simulink model "MTDC_MODEL"  (R2021a)
settings: Solver=ode1  StartTime=0.0  StopTime=3  FixedStep=2e-5  MaxStep=1e-5  RelTol=1e-5  EnableMultiTasking=on
InitFcn:
  | tau_iac=ts_G_iac/4;                                         %Current loop speed
  | wAC=1/tau_iac;                                              %Frequency
  | L1AC=wAC/s;                                                 %Open loop IMC (L) transfer function to obtain a first order after closing the loop
  | Kp_AC=wAC*(Lg_1+La_1/2);                                    %Proportional constant of the controller
  | Ki_AC=wAC*(Rg_1+Ra_1/2);                                    %Integral constant of the controller
  | C_IMC_AC=(Kp_AC*s+Ki_AC)/s;                                 %IMC designed PI controller transfer function
  | TAC=minreal((C_IMC_AC)*G_iac/(1+(C_IMC_AC)*G_iac));         %Closed loop transfer function
  | 
  | tau_Pac=ts_G_P/4;
  | D = TAC*U_ll1;
  | [C_pi,info] = pidtune(D,'PI',1/tau_Pac);
  | Ki_P = C_pi.Ki;
  | 
  | tau_Qac=ts_G_Q/4;
  | [C_piq,info] = pidtune(D,'PI',1/tau_Qac);
  | Ki_Q = C_piq.Ki;
  | 
  | 
  | tau_isum=ts_G_isum/4;                                        %Current loop speed
  | wsum=1/tau_isum;                                             %Frequency
  | L1AC=wsum/s;                                                 %Open loop IMC (L) transfer function to obtain a first order after closing the loop
  | Kp_sum=wsum*(2*La_1);                                        %Proportional constant of the controller
  | Ki_sum=wsum*(2*Ra_1);                                        %Integral constant of the controller
  | C_IMC_sum=(Kp_sum*s+Ki_sum)/s;                               %IMC designed PI controller transfer function
  | 
  | Kp_sum_PR = wc*(2*La_1);
  | Ki_sum_PR = wc*(2*Ra_1);
  | PR = (Kp_sum_PR*s^2 + 2*wc*(Kp_sum_PR+Ki_sum_PR)*s +Kp_sum_PR*w0^2)/(s^2+2*wc*s+w0^2);
  | 
  | 
  | %Energy reference for a converter arm (sum of all the submodule energies)
  | ArmEnergyRef=1/2*Carm*ArmVoltageRef^2;                      %Energy reference for a converter leg
  | LegEnergy=ArmEnergyRef*2;                                   %References for the controllers (DC side)
  | TotalEnergyRef=ArmEnergyRef*6;                              %Reference of the total energy of the converter
  | EnergyDiffabRef=0;                                          %Reference for the energy difference between legs a and b
  | EnergyDiffacRef=0;                                          %Reference for the energy difference between legs b and c
  | 
  | %References for the controllers (AC side)
  | EnergyDiffUpLowRefa=0;                                      %Reference for the energy difference upper and lower arms of phase a
  | EnergyDiffUpLowRefb=0;                                      %Reference for the energy difference upper and lower arms of phase b
  | EnergyDiffUpLowRefc=0;                                      %Reference for the energy difference upper and lower arms of phase c
  |                                                             %Controller design
  | Kpenergy=50;                                                %Proportional gain
  | Kienergy=20;                                                %Integral gain
  | 
  | Kpenergyt=50;                                               %Proportional gain
  | Kienergyt=20;                                               %Integral gain
  | 
  | Q=3;
  | wn=50*2*pi;                                                 %Frequency to eliminate 50 Hz
  | N_50 = tf([1 0 wn^2],[1 2*wn/Q wn^2]);                       %Notch filter 1 design
  | wn=100*2*pi;                                                %Frequency to eliminate 100 Hz
  | N_100 = tf([1 0 wn^2],[1 2*wn/Q wn^2]);                      %Notch filter 2 design
  | Notch=N_50*N_100;                                            %Combination of both notch filters
  | 
  | Ibasedc1= 1000e6/640e3;                 %Nominal current peak DC
  | IsaturationinnerDC1=1.1*Ibasedc1/3;  %Saturation of the DC inner current
  | IsaturationinnerAC1=0.45*Ibasedc1/3; %0.45  %Saturation of the inner current (why edu used 10% - FYI I changed it to 45%)
  | 
  | 
  | ... (+30 lines)
values from neighbouring files (symbols this model uses):
  ArmVoltageRef = 640e3    (= 640000)    [MMC_PARAMETERS.m]
  Cap = 9.5e-3    (= 0.0095)    [MMC_PARAMETERS.m]
  Carm = Cap/N    (= 2.375e-05)    [MMC_PARAMETERS.m]
  f_grid = 50    [MMC_PARAMETERS.m]
  La_1 = 0.15*Zbase_1/2/pi/50    (= 0.0488923985178)    [MMC_PARAMETERS.m]
  Lg_1 = 0.18*Zbase_1/2/pi/50    (= 0.0586708782214)    [MMC_PARAMETERS.m]
  N = 400    [MMC_PARAMETERS.m]
  Ra_1 = 0.01*Zbase_1    (= 1.024)    [MMC_PARAMETERS.m]
  Rg_1 = 0.005*Zbase_1    (= 0.512)    [MMC_PARAMETERS.m]
  S_1 = 1000e6    (= 1000000000)    [MMC_PARAMETERS.m]
  U_ll1 = 320e3    (= 320000)    [MMC_PARAMETERS.m]
  Vdc = 640e3    (= 640000)    [MMC_PARAMETERS.m]
  Vpeak_d1 = U_pnpeak1    [MMC_PARAMETERS.m]
  w0 = 2*pi*50    (= 314.159265359)    [MMC_PARAMETERS.m]
undefined symbols (not defined in the file or in its folder): Kp_Pac, lenght
libraries: spsSeriesRLCBranchLib x80, spsCurrentMeasurementLib x64, spsControlledVoltageSourceLib x36, pid_lib x32, spsVoltageMeasurementLib x32, spsControlledCurrentSourceLib x24, spsParallelRLCBranchLib x20, spsGroundLib x10, powerlib_extras x4, spsDCVoltageSourceLib x4, spspowerguiLib x1
(part 2 of 9)

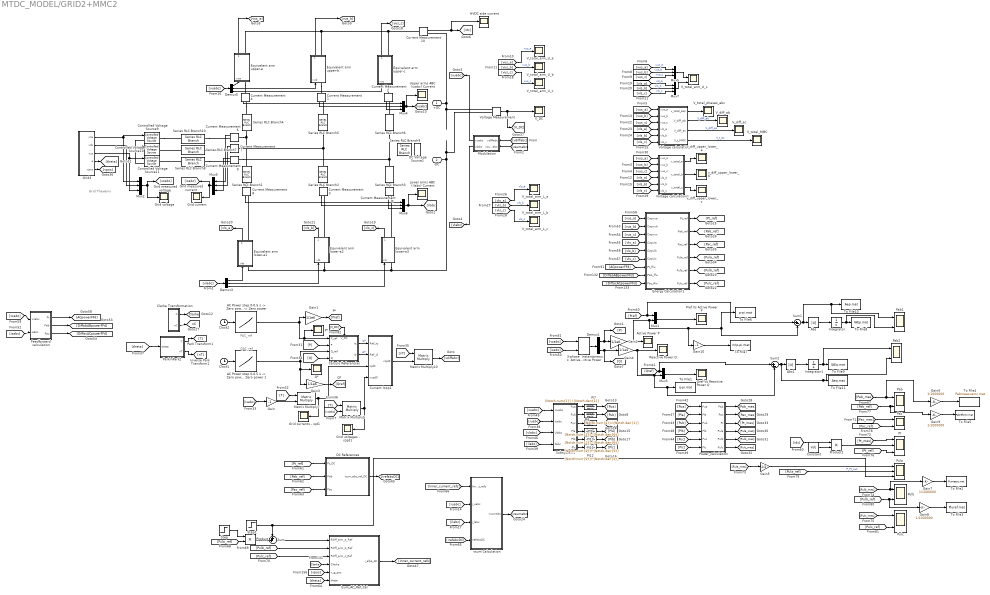
== system MTDC_MODEL/GRID2+MMC2 ==
  note: QAC_ref
  note: Grid Thevenin
  note: PAC_ref
  3-phase  Instantaneous  Active & Reactive Power : powerlib_extras/Measurements/3-phase  Instantaneous  Active & Reactive Power
      settings: SourceProductBaseCode=PS
  "AC Power step 0-0.5 s -> Zero power 0.5-2 s -> Active power injection 2 - 3 s -> Zero power " : Lookup_n-D  NumberOfTableDimensions=1  BreakpointsForDimension1=[0,0.5,2]  Table=[0,100e6,0]  InterpMethod=Flat  RndMeth=Simplest  InputSameDT=on
  "AC Power step 0-0.5 s -> Zero power 0.5-2 s -> Reactive power injection 2 - 3 s -> Zero power 1" : Lookup_n-D  NumberOfTableDimensions=1  BreakpointsForDimension1=[0,1,2]  Table=[0,5e6,0]  InterpMethod=Flat  RndMeth=Simplest  InputSameDT=on
  Abs : Abs
  Abs1 : Abs
  Active Power P : Scope
  Calculo Referencias : Subsystem
      settings: PortSchema="{\"entries\":[{\"content\":{\"sides\":[{\"content\":{\"connectorIds\":[\"In1\",\"In2\",\"In3\",\"In4\"]},\"type\":\"ConnectorPlacement.EquallySpacedRectSide\",\"uuid\":\"f5831c6a-58f5-4c55-8e24-523faf20dc0e\"},{\"content\":{\"connectorIds\":[\"Out1\",\"Out2\"],\"side\":\"RIGHT\"},\"type\":\"ConnectorPlacement.EquallySpacedRectSide\",\"uuid\":\"8e89a825-42f3-407f-8ce2-a529bb4d6e75\"},{\"content\":{\"connectorIds\":[\"In5\"],\"side\":\"TOP\"},\"type\":\"ConnectorPlacement.EquallySpacedRectSide\",\"uuid\":\"db0af466-562a-4a22-9801-d0efcc420c94\"},{\"content\":{\"connectorIds\":[],\"side\":\"BOTTOM\"},\"type\":\"ConnectorPlacement.EquallySpacedRectSide\",\"uuid\":\"e71aeab6-b02a-4177-93b6-e0e9fbfda2d5\"}]},\"type\":\"ConnectorPlacement.EquallySpacedConnector\",\"uuid\":\"54c33138-0c8b-4291-a3b0-05da54bcdffb\"}],\"packageUris\":[\"http://schema.mathworks.com/mf0/Connector/R2020b\"],\"version\":\"1.0\"}"
  "Clarke Transformation " : Subsystem
  Clock1 : Clock
  Clock2 : Clock
  Constant : Constant  Value=Vdc
  Controlled Voltage Source10 : spsControlledVoltageSourceLib/Controlled Voltage Source  Initialize=off  Source_Type=AC  Amplitude=0  Phase=0  Frequency=0  Measurements=None
  Controlled Voltage Source11 : spsControlledVoltageSourceLib/Controlled Voltage Source  Initialize=off  Source_Type=AC  Amplitude=0  Phase=0  Frequency=0  Measurements=None
  Controlled Voltage Source9 : spsControlledVoltageSourceLib/Controlled Voltage Source  Initialize=off  Source_Type=AC  Amplitude=0  Phase=0  Frequency=0  Measurements=None
  Current Measurement{1..10} (10 alike) : spsCurrentMeasurementLib/Current Measurement  PhasorSimulation=off  OutputType=Complex  PSBequivalent=0
  Current loop1 : Subsystem
  DC References : Subsystem
  DC Voltage Source1 : spsDCVoltageSourceLib/DC Voltage Source  Amplitude=Vdc  Measurements=None
  Demux1 : Demux  Outputs=2
  Demux3 : Demux  Outputs=3
  Demux5 : Demux  Outputs=3
  Energy Calculation1 : Subsystem
  Equivalent arm lower-a1 : Subsystem
  Equivalent arm lower-a2 : Subsystem
  Equivalent arm lower-a3 : Subsystem
  Equivalent arm upper-a : Subsystem
  Equivalent arm upper-b : Subsystem
  Equivalent arm upper-c : Subsystem
  Feedforward calculation : Subsystem
  Gain : Gain  Gain=-1
  Gain{1..4} (4 alike) : Gain  Gain=1/1e6
  Gain10 : Gain  Gain=-1
  Gain5 : Gain  Gain=-1/2
  Gain{6..9} (4 alike) : Gain  Gain=1/1000000
  Grid current : Scope
  Grid currents - iqd1 : Scope
  Grid voltage : Scope
  Grid voltages - vzqd1 : Scope
  Grid3 : Subsystem
  HVDC side current : Scope
  Integrator : Integrator
  Integrator1 : Integrator
  Isum_AC_Ref_Cal : Subsystem
  Lower arms ABC (ilabc) Current : Scope
  Matrix Multiply10 : Product  Multiplication=Matrix(*)
  Matrix Multiply5 : Product  Multiplication=Matrix(*)
  Matrix Multiply7 : Product  Multiplication=Matrix(*)
  Modulation : Subsystem
  Mux1 : Mux  Inputs=2
  Mux{2,4..7,9} (6 alike) : Mux  Inputs=3
  Mux3 : Mux  Inputs=2
  P* : Scope
  PI{7..12} (6 alike) : TransferFcn  Numerator=[Notch.num{1}]  Denominator=[Notch.den{1}]
  Pab : Scope  NumInputPorts=2
  Pab1 : Scope  NumInputPorts=2
  Pab2 : Scope  NumInputPorts=2
  Pac : Scope  NumInputPorts=2
  Park/nPark2 : Subsystem
  Power_calculation : Subsystem
  Pref Vs Active Power P : Scope
  Product : Product
  Product1 : Product
  Pt : Scope  NumInputPorts=3
  Pula : Scope  NumInputPorts=3
  Pulb : Scope  NumInputPorts=2
  Pulc : Scope  NumInputPorts=2
  Q* : Scope
  Qref Vs Reactive Power Q : Scope
  Reactive Power Q : Scope
  Series RLC Branch{1..6} (6 alike) : spsSeriesRLCBranchLib/Series RLC Branch  LConnTagsString=__new0  RConnTagsString=__new0  BranchType=RL  Resistance=Ra_1  Inductance=La_1  SetiL0=off  InitialCurrent=0  Capacitance=0  Setx0=off  InitialVoltage=0  Measurements=None
  Series RLC Branch10 : spsSeriesRLCBranchLib/Series RLC Branch  LConnTagsString=__new0  RConnTagsString=__new0  BranchType=RL  Resistance=Rg_1  Inductance=Lg_1  SetiL0=off  InitialCurrent=0  Capacitance=0  Setx0=off  InitialVoltage=0  Measurements=None
  Series RLC Branch7 : spsSeriesRLCBranchLib/Series RLC Branch  LConnTagsString=__new0  RConnTagsString=__new0  BranchType=RL  Resistance=Rg_1  Inductance=Lg_1  SetiL0=off  InitialCurrent=0  Capacitance=0  Setx0=off  InitialVoltage=0  Measurements=None
  Series RLC Branch8 : spsSeriesRLCBranchLib/Series RLC Branch  LConnTagsString=__new0  RConnTagsString=__new0  BranchType=RL  Resistance=Rg_1  Inductance=Lg_1  SetiL0=off  InitialCurrent=0  Capacitance=0  Setx0=off  InitialVoltage=0  Measurements=None
  Series RLC Branch9 : spsSeriesRLCBranchLib/Series RLC Branch  LConnTagsString=__new0  RConnTagsString=__new0  BranchType=C  Resistance=1  Inductance=1e-3  SetiL0=off  InitialCurrent=0  Capacitance=6*Carm  Setx0=off  InitialVoltage=0  Measurements=None
  Step : Step  Time=2.1  Before=1  After=0  SampleTime=0
  Step1 : Step  Time=2.1  After=-1e6  SampleTime=0
  Subsystem1 : Subsystem
  Sum : Sum  Inputs=++|
  Sum1 : Sum  Inputs=|+-
  Sum2 : Sum  Inputs=|+-
  To File1 : ToFile  Filename=q-pi.mat  MatrixName=qsmc  SaveFormat=Timeseries
  To File10 : ToFile  Filename=Aep.mat  MatrixName=Aep  SaveFormat=Timeseries
  To File11 : ToFile  Filename=Aeq.mat  MatrixName=Aeq  SaveFormat=Timeseries
  To File2 : ToFile  Filename=Plumeasu.mat  MatrixName=ans7  SaveFormat=Timeseries
  To File3 : ToFile  Filename=Pluref.mat  MatrixName=ans8  SaveFormat=Timeseries
  To File4 : ToFile  Filename=Pabmeasusmc.mat  MatrixName=ans0002  SaveFormat=Timeseries
  To File5 : ToFile  Filename=Pabrefsmc.mat  MatrixName=ans0001  SaveFormat=Timeseries
  To File6 : ToFile  Filename=p-pi.mat  MatrixName=psmc  SaveFormat=Timeseries
  To File7 : ToFile  Filename=nnp-pi.mat  MatrixName=ans00007  SaveFormat=Timeseries
  To File8 : ToFile  Filename=IAEp.mat  MatrixName=IAEp  SaveFormat=Timeseries
  To File9 : ToFile  Filename=IAEq.mat  MatrixName=IAEq  SaveFormat=Timeseries
  Upper arms ABC (iuabc) Current : Scope
  V_DC : Scope
  V_diff_ab : Scope
  V_diff_ac : Scope
  V_total_MMC : Scope
  V_total_arm_L_a : Scope
  V_total_arm_L_b : Scope
  V_total_arm_L_c : Scope
  V_total_arm_U_L : Scope  NumInputPorts=2
  V_total_arm_U_a : Scope
  V_total_arm_U_b : Scope
  V_total_arm_U_c : Scope
  V_total_phases_abc : Scope
  Voltage Measurement : spsVoltageMeasurementLib/Voltage Measurement  PhasorSimulation=off  OutputType=Complex  PSBequivalent=0
  Voltage calculation : Subsystem
  Voltage calculation1 : Subsystem
  v_diff_upper_lower_a : Scope
  v_diff_upper_lower_b : Scope
  v_diff_upper_lower_c : Scope
  vsum Calculation : Subsystem
  +DC : PMIOPort  Side=Left
  -DC : PMIOPort  Port=2  Side=Left
  tag scope: Clarke=global, nC=global
  wires:
  [V_DC] -> Calculo Referencias/5(V_DC)
  Current Measurement3/1 -> Mux6/2
  [vus_b] -> Energy Calculation1/2(Capvub)
  Energy Calculation1/2(Pab_ref) -> [Pab_ref]
  Voltage calculation1/2(v_total_b) -> v_diff_upper_lower_b/1
  [vus_a] -> Energy Calculation1/1(Capvua)
  Subsystem1/2(Pub) -> PI8/1
  [vls_b] -> Energy Calculation1/5(Capvlb)
  Gain1/1 -> [Pref]
  Current Measurement9/1 -> Mux9/3
  [vls_c] -> V_total_arm_L_c/1  "vls_c"
  Subsystem1/3(Puc) -> PI9/1
  [Pua] -> Power_calculation/1(Pua)
  [vdiffabc] -> Modulation/1(vdiffabc)
  [vzabc] -> 3-phase  Instantaneous  Active & Reactive Power/1
  Current Measurement2/1 -> Mux4/3
  Equivalent arm upper-a/1(v_sum_ua) -> [vus_a]
  [Plc] -> Power_calculation/6(Plc)
  [isabc] -> 3-phase  Instantaneous  Active & Reactive Power/2
  Matrix Multiply10/1 -> [vdiffabc]
  Mux6/1 -> Lower arms ABC (ilabc) Current/1, [ilabc]
  [theta] -> Park/nPark2/1(theta)
  [vls_a] -> Voltage calculation/4(vls_a)
  [P] -> Calculo Referencias/2(P)
  Park/nPark2/2("nT ") -> [nT]
  [nT] -> Matrix Multiply10/1
  Equivalent arm upper-c/1(v_sum_uc) -> [vus_c]
  Gain3/1 -> [Qref]
  Modulation/2(vlabc) -> [vlabc]
  [T] -> Matrix Multiply5/1
  Calculo Referencias/2(id) -> Current loop1/2(Ref_id)  "id*"
  Park/nPark2/1(T) -> [T]
  Voltage calculation/4(V_t_MMC) -> V_total_MMC/1  "V_t_ac"
  [Qref] -> Sum2/1, Mux3/1
  Gain2/1 -> Gain10/1, To File6/1, Sum1/2, Mux1/2, Active Power P/1
  Grid3/1(vza) -> Controlled Voltage Source9/1, Mux2/1
  Current loop1/1(vlqd0) -> Matrix Multiply10/2
  Mux2/1 -> [vzabc], Grid voltage/1
  Equivalent arm lower-a2/1(v_sum_lb) -> [vls_b]
  "AC Power step 0-0.5 s -> Zero power 0.5-2 s -> Reactive power injection 2 - 3 s -> Zero power 1"/1 -> Calculo Referencias/3(Q_ref), Gain3/1, Q*/1
  Equivalent arm lower-a1/1(v_sum_la) -> [vls_a]
  [vus_c] -> V_total_arm_U_c/1  "vus_c"
  [vus_c] -> Mux5/3  "vus_c"
  Voltage calculation/3(V_diff_ac) -> V_diff_ac/1  "V_diff_ac"
  [vus_b] -> V_total_arm_U_b/1  "vus_b"
  Mux3/1 -> Qref Vs Reactive Power Q/1
  [vus_b] -> Mux5/2  "vus_b"
  [vus_c] -> Voltage calculation/3(vus_c)
  [isabc] -> Gain/1
  [vls_b] -> V_total_arm_L_b/1  "vls_b"
  Equivalent arm upper-b/1(v_sum_ub) -> [vus_b]
  [vls_b] -> Mux7/2  "vls_b"
  [vls_a] -> Mux7/1  "vls_a"
  Voltage calculation1/1(v_total_a) -> v_diff_upper_lower_a/1
  [vls_c] -> Voltage calculation/6(vls_c)
  [vus_b] -> Voltage calculation1/2(vus_b)
  [vls_b] -> Voltage calculation1/5(vls_b)
  Constant/1 -> Product1/2
  Demux3/2 -> Equivalent arm lower-a2/1(vlb)
  Clock2/1 -> "AC Power step 0-0.5 s -> Zero power 0.5-2 s -> Active power injection 2 - 3 s -> Zero power "/1
  Matrix Multiply7/1 -> Current loop1/3(iqd0), Grid currents - iqd1/1
  Clock1/1 -> "AC Power step 0-0.5 s -> Zero power 0.5-2 s -> Reactive power injection 2 - 3 s -> Zero power 1"/1
  [vlabc] -> Subsystem1/3(Ulabc)
  [vus_a] -> Mux5/1  "vus_a"
  Gain/1 -> Matrix Multiply7/2
  [vpos] -> Isum_AC_Ref_Cal/5(v_g_pos)
  [Pula_ref] -> Product/2
  Step1/1 -> Pula/3, Sum/1
  Product1/1 -> Pt/2
  [ACpowerFFd] -> Energy Calculation1/7(Pt_ffw)
  [idc] -> Product1/1
  Power_calculation/3(Pt) -> [Pt_mes]
  [DiffabABpowerFFd] -> Energy Calculation1/8(Pab_ffw)
  [vls_a] -> Voltage calculation1/4(vls_a)
  [vus_c] -> Energy Calculation1/3(Capvuc)
  Subsystem1/1(Pua) -> PI7/1
  [Pula_ref] -> Pula/2  "P_PI_out"
  [vls_c] -> Energy Calculation1/6(Capvlc)
  [irefabcDC] -> vsum Calculation/4(irefabcDC)
  [vus_a] -> Voltage calculation1/1(vus_a)
  [Pula_mes] -> Gain5/1
  Mux1/1 -> Pref Vs Active Power P/1
  PI11/1 -> [Plb]
  DC References/1(isum_abc_ref_DC) -> [irefabcDC]
  [Pac_ref] -> DC References/3(Pac)
  Demux1/1 -> [P], Gain2/1
  Step/1 -> Product/1
  [Pub] -> Power_calculation/3(Pub)
  [Pac_mes] -> Pac/1
  [T] -> Matrix Multiply7/1
  Feedforward calculation/2(Pab) -> [DiffabABpowerFFd]
  Voltage Measurement/1 -> [V_DC], V_DC/1
  [vsumabc] -> Modulation/2(vsumabc)
  vsum Calculation/1(vsumabc) -> [vsumabc]
  Power_calculation/2(Pac) -> [Pac_mes]
  PI12/1 -> [Plc]
  [Puc] -> Power_calculation/5(Puc)
  Calculo Referencias/1(iq) -> Current loop1/1(Ref_iq)  "iq*"
  Mux7/1 -> V_total_arm_U_L/2
  Product/1 -> Sum/2
  Modulation/1(vuabc) -> [vuabc]
  Voltage calculation/1(v_total_abc) -> V_total_phases_abc/1
  [vus_a] -> V_total_arm_U_a/1  "vus_a"
  Sum/1 -> Isum_AC_Ref_Cal/1(Pdiff_arm_a_Ref)
  [Pab_ref] -> DC References/2(Pab)
  Power_calculation/5(Pulb) -> [Pulb_mes]
  [Pt_ref] -> Pt/3
  [vus_c] -> Voltage calculation1/3(vus_c)
  [Pref] -> Sum1/1, Mux1/1
  [Pulb_mes] -> Gain7/1, Pulb/1
  PI9/1 -> [Puc]
  Gain4/1 -> Sum2/2, To File1/1, Mux3/2, Reactive Power Q/1
  [vzabc] -> Matrix Multiply5/2
  Energy Calculation1/4(Pula_ref) -> [Pula_ref]
  PI10/1 -> [Pla]
  Power_calculation/6(Pulc) -> [Pulc_mes]
  Gain5/1 -> Pula/1
  Mux5/1 -> V_total_arm_U_L/1
  [Pulc_ref] -> Pulc/2
  [Plb] -> Power_calculation/4(Plb)
  Current Measurement7/1 -> Mux9/2
  PI8/1 -> [Pub]
  "AC Power step 0-0.5 s -> Zero power 0.5-2 s -> Active power injection 2 - 3 s -> Zero power "/1 -> P*/1, Calculo Referencias/1(P_ref), Gain1/1
  [Pulc_mes] -> Pulc/1
  Power_calculation/1(Pab) -> [Pab_mes]
  "Clarke Transformation "/2("nC ") -> [nC]
  Demux5/3 -> Equivalent arm upper-c/1(vuc)
  Energy Calculation1/3(Pac_ref) -> [Pac_ref]
  Mux4/1 -> Upper arms ABC (iuabc) Current/1, [iuabc]
  [Pac_ref] -> Pac/2
  [vls_c] -> Mux7/3  "vls_c"
  Subsystem1/5(Plb) -> PI11/1
  Matrix Multiply5/1 -> Grid voltages - vzqd1/1, Current loop1/4(vzqd0)
  [Pab_ref] -> Gain9/1, Pab/2
  Demux5/1 -> Equivalent arm upper-a/1(vua)
  Grid3/5(vpos) -> [vpos]
  Subsystem1/6(Plc) -> PI12/1
  [Pab_mes] -> Gain6/1, Pab/1
  Grid3/3(vzc) -> Controlled Voltage Source11/1, Mux2/3
  "Clarke Transformation "/1(C) -> [Clarke]
  Subsystem1/4(Pla) -> PI10/1
  [ilabc] -> vsum Calculation/3(i_labc)
  [iuabc] -> vsum Calculation/2(i_uabc)
  [DiffacACpowerFFd] -> Energy Calculation1/9(Pac_ffw)
  [isabc] -> Feedforward calculation/2(isabc)
  [Pulc_ref] -> Isum_AC_Ref_Cal/3(Pdiff_arm_c_Ref)
  [vus_a] -> Voltage calculation/1(vus_a)
  [theta] -> Isum_AC_Ref_Cal/6(theta)
  [vls_b] -> Voltage calculation/5(vls_b)
  [vzabc] -> Feedforward calculation/1(vzabc)
  [Clarke] -> Isum_AC_Ref_Cal/4(Clarke)
  Feedforward calculation/1(Pt) -> [ACpowerFFd]
  Mux9/1 -> [isabc], Grid current/1
  Feedforward calculation/3(Pac) -> [DiffacACpowerFFd]
  Voltage calculation/2(V_diff_ab) -> V_diff_ab/1  "V_diff_ab"
  Demux1/2 -> [Q], Gain4/1
  Current Measurement6/1 -> Mux9/1
  [ilabc] -> Subsystem1/4(Ilabc)
  [Pt_mes] -> Pt/1
  [vus_b] -> Voltage calculation/2(vus_b)
  [Pulb_ref] -> Gain8/1, Pulb/2
  [vlabc] -> Demux3/1
  Energy Calculation1/1(Pt_ref) -> [Pt_ref]
  Voltage calculation1/3(v_total_c) -> v_diff_upper_lower_c/1
  [vls_a] -> V_total_arm_L_a/1  "vls_a"
  Current Measurement4/1 -> Mux4/1
  [vuabc] -> Demux5/1
  Current Measurement1/1 -> Mux4/2
  [iuabc] -> Subsystem1/2(Iuabc)
  [vuabc] -> Subsystem1/1(Uuabc)
  Power_calculation/4(Pula) -> [Pula_mes]
  Demux5/2 -> Equivalent arm upper-b/1(vub)
  PI7/1 -> [Pua]
  [Q] -> Calculo Referencias/4(Q)
  Equivalent arm lower-a3/1(v_sum_lc) -> [vls_c]
  [vls_c] -> Voltage calculation1/6(vls_c)
  Demux3/3 -> Equivalent arm lower-a3/1(vlc)
  3-phase  Instantaneous  Active & Reactive Power/1 -> Demux1/1
  [Pt_ref] -> DC References/1(Pt_DC)
  Isum_AC_Ref_Cal/1(i_albe_AC) -> [Inner_current_refs]
  Energy Calculation1/6(Pulc_ref) -> [Pulc_ref]
  Current Measurement8/1 -> Mux6/1
  Energy Calculation1/5(Pulb_ref) -> [Pulb_ref]
  Current Measurement5/1 -> Mux6/3
  Demux3/1 -> Equivalent arm lower-a1/1(vla)
  [vls_a] -> Energy Calculation1/4(Capvla)
  Grid3/2(vzb) -> Controlled Voltage Source10/1, Mux2/2
  [Pulb_ref] -> Isum_AC_Ref_Cal/2(Pdiff_arm_b_Ref)
  Grid3/4(thetareal) -> [theta]
  [Pla] -> Power_calculation/2(Pla)
  Current Measurement10/1 -> HVDC side current/1, [idc]
  [Inner_current_refs] -> vsum Calculation/1(Inner_current_refs)
  Gain7/1 -> To File2/1
  Gain8/1 -> To File3/1
  Gain6/1 -> To File4/1
  Gain9/1 -> To File5/1
  Gain10/1 -> To File7/1
  Sum1/1 -> Pab1/1, To File10/1, Abs/1
  Abs/1 -> Integrator/1
  Integrator/1 -> Pab1/2, To File8/1
  Integrator1/1 -> Pab2/1, To File9/1
  Abs1/1 -> Integrator1/1
  Sum2/1 -> Pab2/2, To File11/1, Abs1/1
  connections:
  Equivalent arm lower-a1/LConn1 -- Equivalent arm lower-a2/LConn1 -- Voltage Measurement/LConn2 -- -DC/RConn1 -- Equivalent arm lower-a3/LConn1
  Current Measurement6/LConn1 -- Series RLC Branch4/RConn1 -- Series RLC Branch1/LConn1
  Voltage Measurement/LConn1 -- Current Measurement10/RConn1 -- +DC/RConn1
  Controlled Voltage Source10/LConn1 -- Controlled Voltage Source9/LConn1 -- Controlled Voltage Source11/LConn1
  Equivalent arm upper-a/RConn1 -- Current Measurement10/LConn1 -- Equivalent arm upper-c/RConn1 -- Equivalent arm upper-b/RConn1
  Current Measurement7/LConn1 -- Series RLC Branch5/RConn1 -- Series RLC Branch2/LConn1
  Current Measurement9/LConn1 -- Series RLC Branch6/RConn1 -- Series RLC Branch3/LConn1
  Series RLC Branch8/RConn1 -- Current Measurement9/RConn1
  Current Measurement4/RConn1 -- Series RLC Branch4/LConn1
  Series RLC Branch10/RConn1 -- Current Measurement6/RConn1
  Series RLC Branch7/LConn1 -- Controlled Voltage Source10/RConn1
  Equivalent arm lower-a1/RConn1 -- Current Measurement8/RConn1
  Equivalent arm lower-a3/RConn1 -- Current Measurement5/RConn1
  Series RLC Branch3/RConn1 -- Current Measurement5/LConn1
  Series RLC Branch8/LConn1 -- Controlled Voltage Source11/RConn1
  Series RLC Branch7/RConn1 -- Current Measurement7/RConn1
  Series RLC Branch1/RConn1 -- Current Measurement8/LConn1
  Series RLC Branch2/RConn1 -- Current Measurement3/LConn1
  Equivalent arm upper-c/LConn1 -- Current Measurement2/LConn1
  Series RLC Branch6/LConn1 -- Current Measurement2/RConn1
  Equivalent arm lower-a2/RConn1 -- Current Measurement3/RConn1
  Series RLC Branch5/LConn1 -- Current Measurement1/RConn1
  Controlled Voltage Source9/RConn1 -- Series RLC Branch10/LConn1
  Equivalent arm upper-a/LConn1 -- Current Measurement4/LConn1
  Equivalent arm upper-b/LConn1 -- Current Measurement1/LConn1

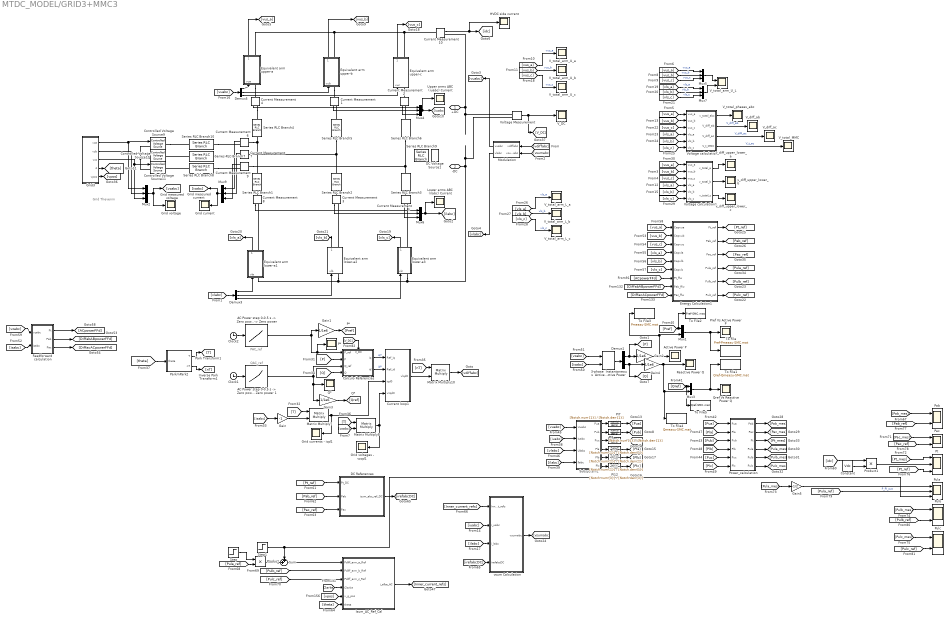
== system MTDC_MODEL/GRID3+MMC3 ==
  note: QAC_ref
  note: Grid Thevenin
  note: PAC_ref
  3-phase  Instantaneous  Active & Reactive Power : powerlib_extras/Measurements/3-phase  Instantaneous  Active & Reactive Power
      settings: SourceProductBaseCode=PS
  "AC Power step 0-0.5 s -> Zero power 0.5-2 s -> Active power injection 2 - 3 s -> Zero power " : Lookup_n-D  NumberOfTableDimensions=1  BreakpointsForDimension1=[0,0.5,2]  Table=[0,-100e6,0]  InterpMethod=Flat  RndMeth=Simplest  InputSameDT=on
  "AC Power step 0-0.5 s -> Zero power 0.5-2 s -> Reactive power injection 2 - 3 s -> Zero power 1" : Lookup_n-D  NumberOfTableDimensions=1  BreakpointsForDimension1=[0,1,2]  Table=[0,-5e6,0]  InterpMethod=Flat  RndMeth=Simplest  InputSameDT=on
  Active Power P : Scope
  Calculo Referencias : Subsystem
      settings: PortSchema="{\"entries\":[{\"content\":{\"sides\":[{\"content\":{\"connectorIds\":[\"In1\",\"In2\",\"In3\",\"In4\"]},\"type\":\"ConnectorPlacement.EquallySpacedRectSide\",\"uuid\":\"f5831c6a-58f5-4c55-8e24-523faf20dc0e\"},{\"content\":{\"connectorIds\":[\"Out1\",\"Out2\"],\"side\":\"RIGHT\"},\"type\":\"ConnectorPlacement.EquallySpacedRectSide\",\"uuid\":\"8e89a825-42f3-407f-8ce2-a529bb4d6e75\"},{\"content\":{\"connectorIds\":[\"In5\"],\"side\":\"TOP\"},\"type\":\"ConnectorPlacement.EquallySpacedRectSide\",\"uuid\":\"db0af466-562a-4a22-9801-d0efcc420c94\"},{\"content\":{\"connectorIds\":[],\"side\":\"BOTTOM\"},\"type\":\"ConnectorPlacement.EquallySpacedRectSide\",\"uuid\":\"e71aeab6-b02a-4177-93b6-e0e9fbfda2d5\"}]},\"type\":\"ConnectorPlacement.EquallySpacedConnector\",\"uuid\":\"54c33138-0c8b-4291-a3b0-05da54bcdffb\"}],\"packageUris\":[\"http://schema.mathworks.com/mf0/Connector/R2020b\"],\"version\":\"1.0\"}"
  Clock1 : Clock
  Clock2 : Clock
  Constant : Constant  Value=Vdc
  Controlled Voltage Source10 : spsControlledVoltageSourceLib/Controlled Voltage Source  Initialize=off  Source_Type=AC  Amplitude=0  Phase=0  Frequency=0  Measurements=None
  Controlled Voltage Source11 : spsControlledVoltageSourceLib/Controlled Voltage Source  Initialize=off  Source_Type=AC  Amplitude=0  Phase=0  Frequency=0  Measurements=None
  Controlled Voltage Source9 : spsControlledVoltageSourceLib/Controlled Voltage Source  Initialize=off  Source_Type=AC  Amplitude=0  Phase=0  Frequency=0  Measurements=None
  Current Measurement{1..10} (10 alike) : spsCurrentMeasurementLib/Current Measurement  PhasorSimulation=off  OutputType=Complex  PSBequivalent=0
  Current loop1 : Subsystem
  DC References : Subsystem
  DC Voltage Source1 : spsDCVoltageSourceLib/DC Voltage Source  Amplitude=Vdc  Measurements=None
  Demux1 : Demux  Outputs=2
  Demux3 : Demux  Outputs=3
  Demux5 : Demux  Outputs=3
  Energy Calculation1 : Subsystem
  Equivalent arm lower-a1 : Subsystem
  Equivalent arm lower-a2 : Subsystem
  Equivalent arm lower-a3 : Subsystem
  Equivalent arm upper-a : Subsystem
  Equivalent arm upper-b : Subsystem
  Equivalent arm upper-c : Subsystem
  Feedforward calculation : Subsystem
  Gain : Gain  Gain=-1
  Gain{1..4} (4 alike) : Gain  Gain=1/1e6
  Gain5 : Gain  Gain=-1/2
  Grid current : Scope
  Grid currents - iqd1 : Scope
  Grid voltage : Scope
  Grid voltages - vzqd1 : Scope
  Grid3 : Subsystem
  HVDC side current : Scope
  Isum_AC_Ref_Cal : Subsystem
  Lower arms ABC (ilabc) Current : Scope
  Matrix Multiply10 : Product  Multiplication=Matrix(*)
  Matrix Multiply5 : Product  Multiplication=Matrix(*)
  Matrix Multiply7 : Product  Multiplication=Matrix(*)
  Modulation : Subsystem
  Mux1 : Mux  Inputs=2
  Mux{2,4..7,9} (6 alike) : Mux  Inputs=3
  Mux3 : Mux  Inputs=2
  P* : Scope
  PI{7..12} (6 alike) : TransferFcn  Numerator=[Notch.num{1}]  Denominator=[Notch.den{1}]
  Pab : Scope  NumInputPorts=2
  Pac : Scope  NumInputPorts=2
  Park/nPark2 : Subsystem
  Power_calculation : Subsystem
  Pref Vs Active Power P : Scope
  Product : Product
  Product1 : Product
  Pt : Scope  NumInputPorts=3
  Pula : Scope  NumInputPorts=3
  Pulb : Scope  NumInputPorts=2
  Pulc : Scope  NumInputPorts=2
  Q* : Scope
  Qref Vs Reactive Power Q : Scope
  Reactive Power Q : Scope
  Series RLC Branch{1..6} (6 alike) : spsSeriesRLCBranchLib/Series RLC Branch  LConnTagsString=__new0  RConnTagsString=__new0  BranchType=RL  Resistance=Ra_1  Inductance=La_1  SetiL0=off  InitialCurrent=0  Capacitance=0  Setx0=off  InitialVoltage=0  Measurements=None
  Series RLC Branch10 : spsSeriesRLCBranchLib/Series RLC Branch  LConnTagsString=__new0  RConnTagsString=__new0  BranchType=RL  Resistance=Rg_1  Inductance=Lg_1  SetiL0=off  InitialCurrent=0  Capacitance=0  Setx0=off  InitialVoltage=0  Measurements=None
  Series RLC Branch7 : spsSeriesRLCBranchLib/Series RLC Branch  LConnTagsString=__new0  RConnTagsString=__new0  BranchType=RL  Resistance=Rg_1  Inductance=Lg_1  SetiL0=off  InitialCurrent=0  Capacitance=0  Setx0=off  InitialVoltage=0  Measurements=None
  Series RLC Branch8 : spsSeriesRLCBranchLib/Series RLC Branch  LConnTagsString=__new0  RConnTagsString=__new0  BranchType=RL  Resistance=Rg_1  Inductance=Lg_1  SetiL0=off  InitialCurrent=0  Capacitance=0  Setx0=off  InitialVoltage=0  Measurements=None
  Series RLC Branch9 : spsSeriesRLCBranchLib/Series RLC Branch  LConnTagsString=__new0  RConnTagsString=__new0  BranchType=C  Resistance=1  Inductance=1e-3  SetiL0=off  InitialCurrent=0  Capacitance=6*Carm  Setx0=off  InitialVoltage=0  Measurements=None
  Step : Step  Time=2.1  Before=1  After=0  SampleTime=0
  Step1 : Step  Time=2.1  After=-1e6  SampleTime=0
  Subsystem1 : Subsystem
  Sum : Sum  Inputs=++|
  To File : ToFile  Filename=Pref-Pmeasu-SMC.mat  MatrixName=ans3  SaveFormat=Timeseries
  To File1 : ToFile  Filename=Qref-Qmeasu-SMC.mat  MatrixName=ans4  SaveFormat=Timeseries
  To File2 : ToFile  Filename=Pref-SMC.mat  MatrixName=ans12  SaveFormat=Timeseries
  To File3 : ToFile  Filename=Pmeasu-SMC.mat  MatrixName=npsmc  SaveFormat=Timeseries
  To File4 : ToFile  Filename=Qmeasu-SMC.mat  MatrixName=nqsmc  SaveFormat=Timeseries
  To File5 : ToFile  Filename=Qref-SMC.mat  MatrixName=ans14  SaveFormat=Timeseries
  Upper arms ABC (iuabc) Current : Scope
  V_DC : Scope
  V_diff_ab : Scope
  V_diff_ac : Scope
  V_total_MMC : Scope
  V_total_arm_L_a : Scope
  V_total_arm_L_b : Scope
  V_total_arm_L_c : Scope
  V_total_arm_U_L : Scope  NumInputPorts=2
  V_total_arm_U_a : Scope
  V_total_arm_U_b : Scope
  V_total_arm_U_c : Scope
  V_total_phases_abc : Scope
  Voltage Measurement : spsVoltageMeasurementLib/Voltage Measurement  PhasorSimulation=off  OutputType=Complex  PSBequivalent=0
  Voltage calculation : Subsystem
  Voltage calculation1 : Subsystem
  v_diff_upper_lower_a : Scope
  v_diff_upper_lower_b : Scope
  v_diff_upper_lower_c : Scope
  vsum Calculation : Subsystem
  +DC : PMIOPort  Side=Left
  -DC : PMIOPort  Port=2  Side=Left
  wires:
  [V_DC] -> Calculo Referencias/5(V_DC)
  Current Measurement3/1 -> Mux6/2
  [vus_b] -> Energy Calculation1/2(Capvub)
  Energy Calculation1/2(Pab_ref) -> [Pab_ref]
  Voltage calculation1/2(v_total_b) -> v_diff_upper_lower_b/1
  [vus_a] -> Energy Calculation1/1(Capvua)
  Subsystem1/2(Pub) -> PI8/1
  [vls_b] -> Energy Calculation1/5(Capvlb)
  Gain1/1 -> [Pref]
  Current Measurement9/1 -> Mux9/3
  [vls_c] -> V_total_arm_L_c/1  "vls_c"
  Subsystem1/3(Puc) -> PI9/1
  [Pua] -> Power_calculation/1(Pua)
  [vdiffabc] -> Modulation/1(vdiffabc)
  [vzabc] -> 3-phase  Instantaneous  Active & Reactive Power/1
  Current Measurement2/1 -> Mux4/3
  Equivalent arm upper-a/1(v_sum_ua) -> [vus_a]
  [Plc] -> Power_calculation/6(Plc)
  [isabc] -> 3-phase  Instantaneous  Active & Reactive Power/2
  Matrix Multiply10/1 -> [vdiffabc]
  Mux6/1 -> Lower arms ABC (ilabc) Current/1, [ilabc]
  [theta] -> Park/nPark2/1(theta)
  [vls_a] -> Voltage calculation/4(vls_a)
  [P] -> Calculo Referencias/2(P)
  Park/nPark2/2("nT ") -> [nT]
  [nT] -> Matrix Multiply10/1
  Equivalent arm upper-c/1(v_sum_uc) -> [vus_c]
  Gain3/1 -> [Qref]
  Modulation/2(vlabc) -> [vlabc]
  [T] -> Matrix Multiply5/1
  Calculo Referencias/2(id) -> Current loop1/2(Ref_id)  "id*"
  Park/nPark2/1(T) -> [T]
  Voltage calculation/4(V_t_MMC) -> V_total_MMC/1  "V_t_ac"
  [Qref] -> To File5/1, Mux3/1
  Gain2/1 -> To File3/1, Mux1/2, Active Power P/1
  Grid3/1(vza) -> Controlled Voltage Source9/1, Mux2/1
  Current loop1/1(vlqd0) -> Matrix Multiply10/2
  Mux2/1 -> [vzabc], Grid voltage/1
  Equivalent arm lower-a2/1(v_sum_lb) -> [vls_b]
  "AC Power step 0-0.5 s -> Zero power 0.5-2 s -> Reactive power injection 2 - 3 s -> Zero power 1"/1 -> Calculo Referencias/3(Q_ref), Gain3/1, Q*/1
  Equivalent arm lower-a1/1(v_sum_la) -> [vls_a]
  [vus_c] -> V_total_arm_U_c/1  "vus_c"
  [vus_c] -> Mux5/3  "vus_c"
  Voltage calculation/3(V_diff_ac) -> V_diff_ac/1  "V_diff_ac"
  [vus_b] -> V_total_arm_U_b/1  "vus_b"
  Mux3/1 -> Qref Vs Reactive Power Q/1, To File1/1
  [vus_b] -> Mux5/2  "vus_b"
  [vus_c] -> Voltage calculation/3(vus_c)
  [isabc] -> Gain/1
  [vls_b] -> V_total_arm_L_b/1  "vls_b"
  Equivalent arm upper-b/1(v_sum_ub) -> [vus_b]
  [vls_b] -> Mux7/2  "vls_b"
  [vls_a] -> Mux7/1  "vls_a"
  Voltage calculation1/1(v_total_a) -> v_diff_upper_lower_a/1
  [vls_c] -> Voltage calculation/6(vls_c)
  [vus_b] -> Voltage calculation1/2(vus_b)
  [vls_b] -> Voltage calculation1/5(vls_b)
  Constant/1 -> Product1/2
  Demux3/2 -> Equivalent arm lower-a2/1(vlb)
  Clock2/1 -> "AC Power step 0-0.5 s -> Zero power 0.5-2 s -> Active power injection 2 - 3 s -> Zero power "/1
  Matrix Multiply7/1 -> Current loop1/3(iqd0), Grid currents - iqd1/1
  Clock1/1 -> "AC Power step 0-0.5 s -> Zero power 0.5-2 s -> Reactive power injection 2 - 3 s -> Zero power 1"/1
  [vlabc] -> Subsystem1/3(Ulabc)
  [vus_a] -> Mux5/1  "vus_a"
  Gain/1 -> Matrix Multiply7/2
  [vpos] -> Isum_AC_Ref_Cal/5(v_g_pos)
  [Pula_ref] -> Product/2
  Step1/1 -> Pula/3, Sum/1
  Product1/1 -> Pt/2
  [ACpowerFFd] -> Energy Calculation1/7(Pt_ffw)
  [idc] -> Product1/1
  Power_calculation/3(Pt) -> [Pt_mes]
  [DiffabABpowerFFd] -> Energy Calculation1/8(Pab_ffw)
  [vls_a] -> Voltage calculation1/4(vls_a)
  [vus_c] -> Energy Calculation1/3(Capvuc)
  Subsystem1/1(Pua) -> PI7/1
  [Pula_ref] -> Pula/2  "P_PI_out"
  [vls_c] -> Energy Calculation1/6(Capvlc)
  [irefabcDC] -> vsum Calculation/4(irefabcDC)
  [vus_a] -> Voltage calculation1/1(vus_a)
  [Pula_mes] -> Gain5/1
  Mux1/1 -> To File/1, Pref Vs Active Power P/1
  PI11/1 -> [Plb]
  DC References/1(isum_abc_ref_DC) -> [irefabcDC]
  [Pac_ref] -> DC References/3(Pac)
  Demux1/1 -> [P], Gain2/1
  Step/1 -> Product/1
  [Pub] -> Power_calculation/3(Pub)
  [Pac_mes] -> Pac/1
  [T] -> Matrix Multiply7/1
  Feedforward calculation/2(Pab) -> [DiffabABpowerFFd]
  Voltage Measurement/1 -> [V_DC], V_DC/1
  [vsumabc] -> Modulation/2(vsumabc)
  vsum Calculation/1(vsumabc) -> [vsumabc]
  Power_calculation/2(Pac) -> [Pac_mes]
  PI12/1 -> [Plc]
  [Puc] -> Power_calculation/5(Puc)
  Calculo Referencias/1(iq) -> Current loop1/1(Ref_iq)  "iq*"
  Mux7/1 -> V_total_arm_U_L/2
  Product/1 -> Sum/2
  Modulation/1(vuabc) -> [vuabc]
  Voltage calculation/1(v_total_abc) -> V_total_phases_abc/1
  [vus_a] -> V_total_arm_U_a/1  "vus_a"
  Sum/1 -> Isum_AC_Ref_Cal/1(Pdiff_arm_a_Ref)
  [Pab_ref] -> DC References/2(Pab)
  Power_calculation/5(Pulb) -> [Pulb_mes]
  [Pt_ref] -> Pt/3
  [vus_c] -> Voltage calculation1/3(vus_c)
  [Pref] -> To File2/1, Mux1/1
  [Pulb_mes] -> Pulb/1
  PI9/1 -> [Puc]
  Gain4/1 -> To File4/1, Mux3/2, Reactive Power Q/1
  [vzabc] -> Matrix Multiply5/2
  Energy Calculation1/4(Pula_ref) -> [Pula_ref]
  PI10/1 -> [Pla]
  Power_calculation/6(Pulc) -> [Pulc_mes]
  Gain5/1 -> Pula/1
  Mux5/1 -> V_total_arm_U_L/1
  [Pulc_ref] -> Pulc/2
  [Plb] -> Power_calculation/4(Plb)
  Current Measurement7/1 -> Mux9/2
  PI8/1 -> [Pub]
  "AC Power step 0-0.5 s -> Zero power 0.5-2 s -> Active power injection 2 - 3 s -> Zero power "/1 -> P*/1, Calculo Referencias/1(P_ref), Gain1/1
  [Pulc_mes] -> Pulc/1
  Power_calculation/1(Pab) -> [Pab_mes]
  Demux5/3 -> Equivalent arm upper-c/1(vuc)
  Energy Calculation1/3(Pac_ref) -> [Pac_ref]
  Mux4/1 -> Upper arms ABC (iuabc) Current/1, [iuabc]
  [Pac_ref] -> Pac/2
  [vls_c] -> Mux7/3  "vls_c"
  Subsystem1/5(Plb) -> PI11/1
  Matrix Multiply5/1 -> Grid voltages - vzqd1/1, Current loop1/4(vzqd0)
  [Pab_ref] -> Pab/2
  Demux5/1 -> Equivalent arm upper-a/1(vua)
  Grid3/5(vpos) -> [vpos]
  Subsystem1/6(Plc) -> PI12/1
  [Pab_mes] -> Pab/1
  Grid3/3(vzc) -> Controlled Voltage Source11/1, Mux2/3
  Subsystem1/4(Pla) -> PI10/1
  [ilabc] -> vsum Calculation/3(i_labc)
  [iuabc] -> vsum Calculation/2(i_uabc)
  [DiffacACpowerFFd] -> Energy Calculation1/9(Pac_ffw)
  [isabc] -> Feedforward calculation/2(isabc)
  [Pulc_ref] -> Isum_AC_Ref_Cal/3(Pdiff_arm_c_Ref)
  [vus_a] -> Voltage calculation/1(vus_a)
  [theta] -> Isum_AC_Ref_Cal/6(theta)
  [vls_b] -> Voltage calculation/5(vls_b)
  [vzabc] -> Feedforward calculation/1(vzabc)
  [Clarke] -> Isum_AC_Ref_Cal/4(Clarke)
  Feedforward calculation/1(Pt) -> [ACpowerFFd]
  Mux9/1 -> [isabc], Grid current/1
  Feedforward calculation/3(Pac) -> [DiffacACpowerFFd]
  Voltage calculation/2(V_diff_ab) -> V_diff_ab/1  "V_diff_ab"
  Demux1/2 -> [Q], Gain4/1
  Current Measurement6/1 -> Mux9/1
  [ilabc] -> Subsystem1/4(Ilabc)
  [Pt_mes] -> Pt/1
  [vus_b] -> Voltage calculation/2(vus_b)
  [Pulb_ref] -> Pulb/2
  [vlabc] -> Demux3/1
  Energy Calculation1/1(Pt_ref) -> [Pt_ref]
  Voltage calculation1/3(v_total_c) -> v_diff_upper_lower_c/1
  [vls_a] -> V_total_arm_L_a/1  "vls_a"
  Current Measurement4/1 -> Mux4/1
  [vuabc] -> Demux5/1
  Current Measurement1/1 -> Mux4/2
  [iuabc] -> Subsystem1/2(Iuabc)
  [vuabc] -> Subsystem1/1(Uuabc)
  Power_calculation/4(Pula) -> [Pula_mes]
  Demux5/2 -> Equivalent arm upper-b/1(vub)
  PI7/1 -> [Pua]
  [Q] -> Calculo Referencias/4(Q)
  Equivalent arm lower-a3/1(v_sum_lc) -> [vls_c]
  [vls_c] -> Voltage calculation1/6(vls_c)
  Demux3/3 -> Equivalent arm lower-a3/1(vlc)
  3-phase  Instantaneous  Active & Reactive Power/1 -> Demux1/1
  [Pt_ref] -> DC References/1(Pt_DC)
  Isum_AC_Ref_Cal/1(i_albe_AC) -> [Inner_current_refs]
  Energy Calculation1/6(Pulc_ref) -> [Pulc_ref]
  Current Measurement8/1 -> Mux6/1
  Energy Calculation1/5(Pulb_ref) -> [Pulb_ref]
  Current Measurement5/1 -> Mux6/3
  Demux3/1 -> Equivalent arm lower-a1/1(vla)
  [vls_a] -> Energy Calculation1/4(Capvla)
  Grid3/2(vzb) -> Controlled Voltage Source10/1, Mux2/2
  [Pulb_ref] -> Isum_AC_Ref_Cal/2(Pdiff_arm_b_Ref)
  Grid3/4(thetareal) -> [theta]
  [Pla] -> Power_calculation/2(Pla)
  Current Measurement10/1 -> HVDC side current/1, [idc]
  [Inner_current_refs] -> vsum Calculation/1(Inner_current_refs)
  connections:
  Equivalent arm lower-a1/LConn1 -- Equivalent arm lower-a2/LConn1 -- Voltage Measurement/LConn2 -- -DC/RConn1 -- Equivalent arm lower-a3/LConn1
  Current Measurement6/LConn1 -- Series RLC Branch4/RConn1 -- Series RLC Branch1/LConn1
  Voltage Measurement/LConn1 -- Current Measurement10/RConn1 -- +DC/RConn1
  Controlled Voltage Source10/LConn1 -- Controlled Voltage Source9/LConn1 -- Controlled Voltage Source11/LConn1
  Equivalent arm upper-a/RConn1 -- Current Measurement10/LConn1 -- Equivalent arm upper-c/RConn1 -- Equivalent arm upper-b/RConn1
  Current Measurement7/LConn1 -- Series RLC Branch5/RConn1 -- Series RLC Branch2/LConn1
  Current Measurement9/LConn1 -- Series RLC Branch6/RConn1 -- Series RLC Branch3/LConn1
  Series RLC Branch8/RConn1 -- Current Measurement9/RConn1
  Current Measurement4/RConn1 -- Series RLC Branch4/LConn1
  Series RLC Branch10/RConn1 -- Current Measurement6/RConn1
  Series RLC Branch7/LConn1 -- Controlled Voltage Source10/RConn1
  Equivalent arm lower-a1/RConn1 -- Current Measurement8/RConn1
  Equivalent arm lower-a3/RConn1 -- Current Measurement5/RConn1
  Series RLC Branch3/RConn1 -- Current Measurement5/LConn1
  Series RLC Branch8/LConn1 -- Controlled Voltage Source11/RConn1
  Series RLC Branch7/RConn1 -- Current Measurement7/RConn1
  Series RLC Branch1/RConn1 -- Current Measurement8/LConn1
  Series RLC Branch2/RConn1 -- Current Measurement3/LConn1
  Equivalent arm upper-c/LConn1 -- Current Measurement2/LConn1
  Series RLC Branch6/LConn1 -- Current Measurement2/RConn1
  Equivalent arm lower-a2/RConn1 -- Current Measurement3/RConn1
  Series RLC Branch5/LConn1 -- Current Measurement1/RConn1
  Controlled Voltage Source9/RConn1 -- Series RLC Branch10/LConn1
  Equivalent arm upper-a/LConn1 -- Current Measurement4/LConn1
  Equivalent arm upper-b/LConn1 -- Current Measurement1/LConn1
